simulink model "case4"  (R2024b)
settings: Solver=FixedStepAuto  StartTime=0  StopTime=1  FixedStep=1e-7  RelTol=1e-3
values from neighbouring files (symbols this model uses):
  SG_D_1_D = 0.01056    [IEEE9_case_parameters.m]    (also in case1_parameters.m; case2_parameters.m; case3_parameters.m; case4_parameters.m)
  SG_D_1_EnableSaturation = 0    [IEEE9_case_parameters.m]    (also in case1_parameters.m; case2_parameters.m; case3_parameters.m; case4_parameters.m)
  SG_D_1_f0 = 60    [IEEE9_case_parameters.m]    (also in case1_parameters.m; case2_parameters.m; case3_parameters.m; case4_parameters.m)
  SG_D_1_H = 7.5    [IEEE9_case_parameters.m]    (also in case1_parameters.m; case2_parameters.m; case3_parameters.m; case4_parameters.m)
  SG_D_1_K_A = 20    [IEEE9_case_parameters.m]    (also in case1_parameters.m; case2_parameters.m; case3_parameters.m; case4_parameters.m)
  SG_D_1_K_E = 1.000000e+1    (= 10)    [IEEE9_case_parameters.m]    (also in case1_parameters.m; case2_parameters.m; case3_parameters.m; case4_parameters.m)
  SG_D_1_K_F = 2.363    [IEEE9_case_parameters.m]    (also in case1_parameters.m; case2_parameters.m; case3_parameters.m; case4_parameters.m)
  SG_D_1_K_s = 0.5    [IEEE9_case_parameters.m]    (also in case1_parameters.m = 5; case2_parameters.m = 5; case3_parameters.m = 5; case4_parameters.m = 5)
  SG_D_1_R_a = 0.001088    [IEEE9_case_parameters.m]    (also in case1_parameters.m; case2_parameters.m; case3_parameters.m; case4_parameters.m)
  SG_D_1_S_A = 1    [IEEE9_case_parameters.m]    (also in case1_parameters.m; case2_parameters.m; case3_parameters.m; case4_parameters.m)
  SG_D_1_S_B = 0.103    [IEEE9_case_parameters.m]    (also in case1_parameters.m; case2_parameters.m; case3_parameters.m; case4_parameters.m)
  SG_D_1_S_N = 10.659857    [IEEE9_case_parameters.m]    (also in case1_parameters.m; case2_parameters.m; case3_parameters.m; case4_parameters.m)
  SG_D_1_SpeedPara = 200    [IEEE9_case_parameters.m]    (also in case1_parameters.m; case2_parameters.m; case3_parameters.m; case4_parameters.m)
  SG_D_1_T_0 = 0.720173    [IEEE9_case_parameters.m]    (also in case1_parameters.m = 0.755522; case2_parameters.m = 0.808931; case3_parameters.m = 0.869402; case4_parameters.m = 0.729316)
  SG_D_1_T_1 = 0.3    [IEEE9_case_parameters.m]    (also in case1_parameters.m; case2_parameters.m; case3_parameters.m; case4_parameters.m)
  SG_D_1_T_2 = 0.05    [IEEE9_case_parameters.m]    (also in case1_parameters.m; case2_parameters.m; case3_parameters.m; case4_parameters.m)
  SG_D_1_T_3 = 0.02    [IEEE9_case_parameters.m]    (also in case1_parameters.m; case2_parameters.m; case3_parameters.m; case4_parameters.m)
  SG_D_1_T_4 = 0.005    [IEEE9_case_parameters.m]    (also in case1_parameters.m; case2_parameters.m; case3_parameters.m; case4_parameters.m)
  SG_D_1_T_A = 0.02    [IEEE9_case_parameters.m]    (also in case1_parameters.m; case2_parameters.m; case3_parameters.m; case4_parameters.m)
  SG_D_1_T_dd = 8.000000e+0    (= 8)    [IEEE9_case_parameters.m]    (also in case1_parameters.m; case2_parameters.m; case3_parameters.m; case4_parameters.m)
  SG_D_1_T_ddd = 0.04    [IEEE9_case_parameters.m]    (also in case1_parameters.m; case2_parameters.m; case3_parameters.m; case4_parameters.m)
  SG_D_1_T_E = 0.314    [IEEE9_case_parameters.m]    (also in case1_parameters.m; case2_parameters.m; case3_parameters.m; case4_parameters.m)
  SG_D_1_T_F = 0.35    [IEEE9_case_parameters.m]    (also in case1_parameters.m; case2_parameters.m; case3_parameters.m; case4_parameters.m)
  SG_D_1_T_qd = 0.8    [IEEE9_case_parameters.m]    (also in case1_parameters.m; case2_parameters.m; case3_parameters.m; case4_parameters.m)
  SG_D_1_T_qdd = 0.02    [IEEE9_case_parameters.m]    (also in case1_parameters.m; case2_parameters.m; case3_parameters.m; case4_parameters.m)
  SG_D_1_T_speed = 0.1    [IEEE9_case_parameters.m]    (also in case1_parameters.m = 200; case2_parameters.m = 200; case3_parameters.m = 200; case4_parameters.m = 200)
  SG_D_1_T_w = 0.5    [IEEE9_case_parameters.m]    (also in case1_parameters.m; case2_parameters.m; case3_parameters.m; case4_parameters.m)
  SG_D_1_V_ref = 1.990276    [IEEE9_case_parameters.m]    (also in case1_parameters.m = 2.042296; case2_parameters.m = 2.051388; case3_parameters.m = 2.089584; case4_parameters.m = 2.01845)
  SG_D_1_w_ref = 376.991118    [IEEE9_case_parameters.m]    (also in case1_parameters.m; case2_parameters.m; case3_parameters.m; case4_parameters.m)
  SG_D_1_wb = 6.000000e+1    (= 60)    [IEEE9_case_parameters.m]    (also in case1_parameters.m; case2_parameters.m; case3_parameters.m; case4_parameters.m)
  SG_D_1_x_d = 1.9    [IEEE9_case_parameters.m]    (also in case1_parameters.m; case2_parameters.m; case3_parameters.m; case4_parameters.m)
  SG_D_1_x_dd = 0.302    [IEEE9_case_parameters.m]    (also in case1_parameters.m; case2_parameters.m; case3_parameters.m; case4_parameters.m)
  SG_D_1_x_ddd = 0.204    [IEEE9_case_parameters.m]    (also in case1_parameters.m; case2_parameters.m; case3_parameters.m; case4_parameters.m)
  SG_D_1_x_l = 0.05    [IEEE9_case_parameters.m]    (also in case1_parameters.m; case2_parameters.m; case3_parameters.m; case4_parameters.m)
  SG_D_1_x_q = 1.3    [IEEE9_case_parameters.m]    (also in case1_parameters.m; case2_parameters.m; case3_parameters.m; case4_parameters.m)
  SG_D_1_x_qd = 0.5    [IEEE9_case_parameters.m]    (also in case1_parameters.m; case2_parameters.m; case3_parameters.m; case4_parameters.m)
  SG_D_1_x_qdd = 0.3    [IEEE9_case_parameters.m]    (also in case1_parameters.m; case2_parameters.m; case3_parameters.m; case4_parameters.m)
  SG_D_2_D = 0.02    [IEEE9_case_parameters.m]    (also in case1_parameters.m; case2_parameters.m; case3_parameters.m; case4_parameters.m)
  SG_D_2_EnableSaturation = 0    [IEEE9_case_parameters.m]    (also in case1_parameters.m; case2_parameters.m; case3_parameters.m; case4_parameters.m)
  SG_D_2_f0 = 60    [IEEE9_case_parameters.m]    (also in case1_parameters.m; case2_parameters.m; case3_parameters.m; case4_parameters.m)
  SG_D_2_H = 8.000000e+0    (= 8)    [IEEE9_case_parameters.m]    (also in case1_parameters.m; case2_parameters.m; case3_parameters.m; case4_parameters.m)
  SG_D_2_K_A = 20    [IEEE9_case_parameters.m]    (also in case1_parameters.m; case2_parameters.m; case3_parameters.m; case4_parameters.m)
  SG_D_2_K_E = 1.000000e+1    (= 10)    [IEEE9_case_parameters.m]    (also in case1_parameters.m; case2_parameters.m; case3_parameters.m; case4_parameters.m)
  SG_D_2_K_F = 2.363    [IEEE9_case_parameters.m]    (also in case1_parameters.m; case2_parameters.m; case3_parameters.m; case4_parameters.m)
  SG_D_2_K_s = 0.5    [IEEE9_case_parameters.m]    (also in case1_parameters.m = 4; case2_parameters.m = 4; case3_parameters.m = 4; case4_parameters.m = 4)
  SG_D_2_R_a = 0.001088    [IEEE9_case_parameters.m]    (also in case1_parameters.m; case2_parameters.m; case3_parameters.m; case4_parameters.m)
  SG_D_2_S_A = 1    [IEEE9_case_parameters.m]    (also in case1_parameters.m; case2_parameters.m; case3_parameters.m; case4_parameters.m)
  SG_D_2_S_B = 0.103    [IEEE9_case_parameters.m]    (also in case1_parameters.m; case2_parameters.m; case3_parameters.m; case4_parameters.m)
  SG_D_2_S_N = 10.659857    [IEEE9_case_parameters.m]    (also in case1_parameters.m; case2_parameters.m; case3_parameters.m; case4_parameters.m)
  SG_D_2_SpeedPara = 200    [IEEE9_case_parameters.m]    (also in case1_parameters.m; case2_parameters.m; case3_parameters.m; case4_parameters.m)
  SG_D_2_T_0 = 1.632913    [IEEE9_case_parameters.m]    (also in case1_parameters.m = 1.632925; case2_parameters.m = 1.632915; case3_parameters.m = 1.632914; case4_parameters.m = 1.632927)
  SG_D_2_T_1 = 0.2    [IEEE9_case_parameters.m]    (also in case1_parameters.m; case2_parameters.m; case3_parameters.m; case4_parameters.m)
  SG_D_2_T_2 = 0.05    [IEEE9_case_parameters.m]    (also in case1_parameters.m; case2_parameters.m; case3_parameters.m; case4_parameters.m)
  SG_D_2_T_3 = 0.02    [IEEE9_case_parameters.m]    (also in case1_parameters.m; case2_parameters.m; case3_parameters.m; case4_parameters.m)
  SG_D_2_T_4 = 0.005    [IEEE9_case_parameters.m]    (also in case1_parameters.m; case2_parameters.m; case3_parameters.m; case4_parameters.m)
  SG_D_2_T_A = 0.02    [IEEE9_case_parameters.m]    (also in case1_parameters.m; case2_parameters.m; case3_parameters.m; case4_parameters.m)
  SG_D_2_T_dd = 7.9    [IEEE9_case_parameters.m]    (also in case1_parameters.m; case2_parameters.m; case3_parameters.m; case4_parameters.m)
  SG_D_2_T_ddd = 0.04    [IEEE9_case_parameters.m]    (also in case1_parameters.m; case2_parameters.m; case3_parameters.m; case4_parameters.m)
  SG_D_2_T_E = 0.314    [IEEE9_case_parameters.m]    (also in case1_parameters.m; case2_parameters.m; case3_parameters.m; case4_parameters.m)
  SG_D_2_T_F = 0.35    [IEEE9_case_parameters.m]    (also in case1_parameters.m; case2_parameters.m; case3_parameters.m; case4_parameters.m)
  SG_D_2_T_qd = 0.8    [IEEE9_case_parameters.m]    (also in case1_parameters.m; case2_parameters.m; case3_parameters.m; case4_parameters.m)
  SG_D_2_T_qdd = 0.015    [IEEE9_case_parameters.m]    (also in case1_parameters.m; case2_parameters.m; case3_parameters.m; case4_parameters.m)
  SG_D_2_T_speed = 0.1    [IEEE9_case_parameters.m]    (also in case1_parameters.m = 150; case2_parameters.m = 150; case3_parameters.m = 150; case4_parameters.m = 150)
  SG_D_2_T_w = 0.35    [IEEE9_case_parameters.m]    (also in case1_parameters.m; case2_parameters.m; case3_parameters.m; case4_parameters.m)
  SG_D_2_V_ref = 2.58547    [IEEE9_case_parameters.m]    (also in case1_parameters.m = 2.597896; case2_parameters.m = 2.587136; case3_parameters.m = 2.586042; case4_parameters.m = 2.599679)
  SG_D_2_w_ref = 376.991118    [IEEE9_case_parameters.m]    (also in case1_parameters.m; case2_parameters.m; case3_parameters.m; case4_parameters.m)
  SG_D_2_wb = 6.000000e+1    (= 60)    [IEEE9_case_parameters.m]    (also in case1_parameters.m; case2_parameters.m; case3_parameters.m; case4_parameters.m)
  SG_D_2_x_d = 1.8    [IEEE9_case_parameters.m]    (also in case1_parameters.m; case2_parameters.m; case3_parameters.m; case4_parameters.m)
  SG_D_2_x_dd = 0.302    [IEEE9_case_parameters.m]    (also in case1_parameters.m; case2_parameters.m; case3_parameters.m; case4_parameters.m)
  SG_D_2_x_ddd = 0.204    [IEEE9_case_parameters.m]    (also in case1_parameters.m; case2_parameters.m; case3_parameters.m; case4_parameters.m)
  SG_D_2_x_l = 0.05    [IEEE9_case_parameters.m]    (also in case1_parameters.m; case2_parameters.m; case3_parameters.m; case4_parameters.m)
  SG_D_2_x_q = 1.25    [IEEE9_case_parameters.m]    (also in case1_parameters.m; case2_parameters.m; case3_parameters.m; case4_parameters.m)
  SG_D_2_x_qd = 0.5    [IEEE9_case_parameters.m]    (also in case1_parameters.m; case2_parameters.m; case3_parameters.m; case4_parameters.m)
  SG_D_2_x_qdd = 0.3    [IEEE9_case_parameters.m]    (also in case1_parameters.m; case2_parameters.m; case3_parameters.m; case4_parameters.m)
  SG_D_3_D = 0.02    [IEEE9_case_parameters.m]    (also in case1_parameters.m; case2_parameters.m; case3_parameters.m; case4_parameters.m)
  SG_D_3_EnableSaturation = 0    [IEEE9_case_parameters.m]    (also in case1_parameters.m; case2_parameters.m; case3_parameters.m; case4_parameters.m)
  SG_D_3_f0 = 60    [IEEE9_case_parameters.m]    (also in case1_parameters.m; case2_parameters.m; case3_parameters.m; case4_parameters.m)
  SG_D_3_H = 7.7    [IEEE9_case_parameters.m]    (also in case1_parameters.m; case2_parameters.m; case3_parameters.m; case4_parameters.m)
  SG_D_3_K_A = 20    [IEEE9_case_parameters.m]    (also in case1_parameters.m; case2_parameters.m; case3_parameters.m; case4_parameters.m)
  SG_D_3_K_E = 1.000000e+1    (= 10)    [IEEE9_case_parameters.m]    (also in case1_parameters.m; case2_parameters.m; case3_parameters.m; case4_parameters.m)
  SG_D_3_K_F = 2.363    [IEEE9_case_parameters.m]    (also in case1_parameters.m; case2_parameters.m; case3_parameters.m; case4_parameters.m)
  SG_D_3_K_s = 0.2    [IEEE9_case_parameters.m]    (also in case1_parameters.m = 2; case2_parameters.m = 2; case3_parameters.m = 2; case4_parameters.m = 2)
  SG_D_3_R_a = 0.001088    [IEEE9_case_parameters.m]    (also in case1_parameters.m; case2_parameters.m; case3_parameters.m; case4_parameters.m)
  SG_D_3_S_A = 1    [IEEE9_case_parameters.m]    (also in case1_parameters.m; case2_parameters.m; case3_parameters.m; case4_parameters.m)
  SG_D_3_S_B = 0.103    [IEEE9_case_parameters.m]    (also in case1_parameters.m; case2_parameters.m; case3_parameters.m; case4_parameters.m)
  SG_D_3_S_N = 10.659857    [IEEE9_case_parameters.m]    (also in case1_parameters.m; case2_parameters.m; case3_parameters.m; case4_parameters.m)
  SG_D_3_SpeedPara = 200    [IEEE9_case_parameters.m]    (also in case1_parameters.m; case2_parameters.m; case3_parameters.m; case4_parameters.m)
  SG_D_3_T_0 = 0.850788    [IEEE9_case_parameters.m]    (also in case1_parameters.m = 0.850786; case2_parameters.m = 0.850787; case3_parameters.m; case4_parameters.m = 0.850786)
  SG_D_3_T_1 = 0.2    [IEEE9_case_parameters.m]    (also in case1_parameters.m; case2_parameters.m; case3_parameters.m; case4_parameters.m)
  SG_D_3_T_2 = 0.05    [IEEE9_case_parameters.m]    (also in case1_parameters.m; case2_parameters.m; case3_parameters.m; case4_parameters.m)
  SG_D_3_T_3 = 0.02    [IEEE9_case_parameters.m]    (also in case1_parameters.m; case2_parameters.m; case3_parameters.m; case4_parameters.m)
  SG_D_3_T_4 = 0.005    [IEEE9_case_parameters.m]    (also in case1_parameters.m; case2_parameters.m; case3_parameters.m; case4_parameters.m)
  SG_D_3_T_A = 0.02    [IEEE9_case_parameters.m]    (also in case1_parameters.m; case2_parameters.m; case3_parameters.m; case4_parameters.m)
  SG_D_3_T_dd = 8.1    [IEEE9_case_parameters.m]    (also in case1_parameters.m; case2_parameters.m; case3_parameters.m; case4_parameters.m)
  SG_D_3_T_ddd = 0.04    [IEEE9_case_parameters.m]    (also in case1_parameters.m; case2_parameters.m; case3_parameters.m; case4_parameters.m)
  SG_D_3_T_E = 0.314    [IEEE9_case_parameters.m]    (also in case1_parameters.m; case2_parameters.m; case3_parameters.m; case4_parameters.m)
  SG_D_3_T_F = 0.35    [IEEE9_case_parameters.m]    (also in case1_parameters.m; case2_parameters.m; case3_parameters.m; case4_parameters.m)
  SG_D_3_T_qd = 0.8    [IEEE9_case_parameters.m]    (also in case1_parameters.m; case2_parameters.m; case3_parameters.m; case4_parameters.m)
  SG_D_3_T_qdd = 0.015    [IEEE9_case_parameters.m]    (also in case1_parameters.m; case2_parameters.m; case3_parameters.m; case4_parameters.m)
  SG_D_3_T_speed = 0.1    [IEEE9_case_parameters.m]    (also in case1_parameters.m = 180; case2_parameters.m = 180; case3_parameters.m = 180; case4_parameters.m = 180)
  SG_D_3_T_w = 0.4    [IEEE9_case_parameters.m]    (also in case1_parameters.m; case2_parameters.m; case3_parameters.m; case4_parameters.m)
  SG_D_3_V_ref = 1.892727    [IEEE9_case_parameters.m]    (also in case1_parameters.m = 1.906439; case2_parameters.m = 1.895535; case3_parameters.m = 1.892105; case4_parameters.m = 1.906598)
  SG_D_3_w_ref = 376.991118    [IEEE9_case_parameters.m]    (also in case1_parameters.m; case2_parameters.m; case3_parameters.m; case4_parameters.m)
  SG_D_3_wb = 6.000000e+1    (= 60)    [IEEE9_case_parameters.m]    (also in case1_parameters.m; case2_parameters.m; case3_parameters.m; case4_parameters.m)
  SG_D_3_x_d = 1.85    [IEEE9_case_parameters.m]    (also in case1_parameters.m; case2_parameters.m; case3_parameters.m; case4_parameters.m)
  SG_D_3_x_dd = 0.302    [IEEE9_case_parameters.m]    (also in case1_parameters.m; case2_parameters.m; case3_parameters.m; case4_parameters.m)
  SG_D_3_x_ddd = 0.204    [IEEE9_case_parameters.m]    (also in case1_parameters.m; case2_parameters.m; case3_parameters.m; case4_parameters.m)
  SG_D_3_x_l = 0.05    [IEEE9_case_parameters.m]    (also in case1_parameters.m; case2_parameters.m; case3_parameters.m; case4_parameters.m)
  SG_D_3_x_q = 1.2    [IEEE9_case_parameters.m]    (also in case1_parameters.m; case2_parameters.m; case3_parameters.m; case4_parameters.m)
  SG_D_3_x_qd = 0.5    [IEEE9_case_parameters.m]    (also in case1_parameters.m; case2_parameters.m; case3_parameters.m; case4_parameters.m)
  SG_D_3_x_qdd = 0.3    [IEEE9_case_parameters.m]    (also in case1_parameters.m; case2_parameters.m; case3_parameters.m; case4_parameters.m)
(part 2 of 12)

== system case4/SG_D_2 ==
  v_d_SG_D_2 : Inport
  v_q_SG_D_2 : Inport  Port=2
  E_fd_SG_D_2 : Integrator  InitialCondition=3.199358804894044
  Px_1_SG_D_2 : Integrator  InitialCondition=0.0
  Px_2_SG_D_2 : Integrator  InitialCondition=0.0
  Px_3_SG_D_2 : Integrator  InitialCondition=-1.0252237820631645e-24
  R_f_SG_D_2 : Integrator  InitialCondition=21.60024244561322
  T_e_SG_D_2_block : Subsystem
  T_m_SG_D_2 : Integrator  InitialCondition=1.632927067566547
  V_f_SG_D_2 : Integrator  InitialCondition=31.993588048940442
  d_E_fd_SG_D_2_block : Subsystem
  d_Px_1_SG_D_2_block : Subsystem
  d_Px_2_SG_D_2_block : Subsystem
  d_Px_3_SG_D_2_block : Subsystem
  d_R_f_SG_D_2_block : Subsystem
  d_T_m_SG_D_2_block : Subsystem
  d_V_f_SG_D_2_block : Subsystem
  d_psi_1d_SG_D_2_block : Subsystem
  d_psi_d_SG_D_2_block : Subsystem
  d_psi_fd_SG_D_2_block : Subsystem
  d_psi_gq_SG_D_2_block : Subsystem
  d_psi_kq_SG_D_2_block : Subsystem
  d_psi_q_SG_D_2_block : Subsystem
  d_theta_SG_D_2_block : Subsystem
  d_w_SG_D_2_block : Subsystem
  i_d_SG_D_2_block : Subsystem
  i_q_SG_D_2_block : Subsystem
  psi_1d_SG_D_2 : Integrator  InitialCondition=0.5921734460690405
  psi_d_SG_D_2 : Integrator  InitialCondition=0.5176824358168975
  psi_fd_SG_D_2 : Integrator  InitialCondition=0.9676081377398411
  psi_gq_SG_D_2 : Integrator  InitialCondition=0.514587004954726
  psi_kq_SG_D_2 : Integrator  InitialCondition=-0.8233392079275615
  psi_q_SG_D_2 : Integrator  InitialCondition=-0.8576450082578766
  theta_SG_D_2 : Integrator  InitialCondition=1.203497719672738
  theta_SG_D_2_out_block : Subsystem
  w_SG_D_2 : Integrator  InitialCondition=376.99111843077515
  w_SG_D_2_out_block : Subsystem
  i_d_SG_D_2 : Outport
  i_q_SG_D_2 : Outport  Port=2
  T_e_SG_D_2 : Outport  Port=3
  w_SG_D_2_out : Outport  Port=4
  theta_SG_D_2_out : Outport  Port=5
  wires:
  T_e_SG_D_2_block/1(Blockout_T_e_SG_D_2_aeb34) -> T_e_SG_D_2/1
  d_Px_2_SG_D_2_block/1(Blockout_d_Px_2_SG_D_2_a31a2) -> Px_2_SG_D_2/1
  d_T_m_SG_D_2_block/1(Blockout_d_T_m_SG_D_2_16fb0) -> T_m_SG_D_2/1
  w_SG_D_2/1 -> d_w_SG_D_2_block/1(State_w_SG_D_2_24507), d_psi_d_SG_D_2_block/9(State_w_SG_D_2_062a2), d_V_f_SG_D_2_block/13(State_w_SG_D_2_1f752), d_psi_q_SG_D_2_block/9(State_w_SG_D_2_85500), d_T_m_SG_D_2_block/1(State_w_SG_D_2_20fb2), d_theta_SG_D_2_block/1(State_w_SG_D_2_83554), d_Px_2_SG_D_2_block/4(State_w_SG_D_2_251c8), d_Px_3_SG_D_2_block/6(State_w_SG_D_2_cceda), d_Px_1_SG_D_2_block/2(State_w_SG_D_2_89096), w_SG_D_2_out_block/1(State_w_SG_D_2_49837), d_V_f_SG_D_2_block/8(State_w_SG_D_2_d8cc8)
  psi_q_SG_D_2/1 -> d_psi_d_SG_D_2_block/8(State_psi_q_SG_D_2_4ef81), d_psi_gq_SG_D_2_block/6(State_psi_q_SG_D_2_42d41), d_psi_gq_SG_D_2_block/9(State_psi_q_SG_D_2_df93d), d_psi_q_SG_D_2_block/3(State_psi_q_SG_D_2_7ccc9), d_psi_kq_SG_D_2_block/5(State_psi_q_SG_D_2_06ac6), d_w_SG_D_2_block/6(State_psi_q_SG_D_2_486c0), d_w_SG_D_2_block/7(State_psi_q_SG_D_2_c0a51), i_d_SG_D_2_block/3(State_psi_q_SG_D_2_d9bdd), i_q_SG_D_2_block/3(State_psi_q_SG_D_2_089b8), d_V_f_SG_D_2_block/7(State_psi_q_SG_D_2_113af), T_e_SG_D_2_block/4(State_psi_q_SG_D_2_38137), T_e_SG_D_2_block/5(State_psi_q_SG_D_2_ed317), d_V_f_SG_D_2_block/11(State_psi_q_SG_D_2_905ca)
  w_SG_D_2_out_block/1(Blockout_w_SG_D_2_out_2aeb7) -> w_SG_D_2_out/1
  T_m_SG_D_2/1 -> d_T_m_SG_D_2_block/2(State_T_m_SG_D_2_247d7), d_w_SG_D_2_block/2(State_T_m_SG_D_2_a1094)
  d_theta_SG_D_2_block/1(Blockout_d_theta_SG_D_2_36a6f) -> theta_SG_D_2/1
  d_Px_1_SG_D_2_block/1(Blockout_d_Px_1_SG_D_2_f7300) -> Px_1_SG_D_2/1
  d_Px_3_SG_D_2_block/1(Blockout_d_Px_3_SG_D_2_a07c3) -> Px_3_SG_D_2/1
  Px_2_SG_D_2/1 -> d_Px_2_SG_D_2_block/1(State_Px_2_SG_D_2_0c5e7), d_Px_3_SG_D_2_block/2(State_Px_2_SG_D_2_117c1), d_Px_3_SG_D_2_block/3(State_Px_2_SG_D_2_e0625)
  theta_SG_D_2/1 -> d_psi_d_SG_D_2_block/7(State_theta_SG_D_2_7f4d5), i_d_SG_D_2_block/8(State_theta_SG_D_2_c3678), i_q_SG_D_2_block/4(State_theta_SG_D_2_9d528), d_psi_q_SG_D_2_block/7(State_theta_SG_D_2_47b3e), i_q_SG_D_2_block/8(State_theta_SG_D_2_f85ec), i_d_SG_D_2_block/4(State_theta_SG_D_2_d89e5), theta_SG_D_2_out_block/1(State_theta_SG_D_2_ce1d4), d_psi_q_SG_D_2_block/5(State_theta_SG_D_2_14fc9), d_psi_d_SG_D_2_block/5(State_theta_SG_D_2_f56a2)
  i_d_SG_D_2_block/1(Blockout_i_d_SG_D_2_51594) -> i_d_SG_D_2/1
  psi_d_SG_D_2/1 -> d_psi_fd_SG_D_2_block/6(State_psi_d_SG_D_2_a4384), d_psi_fd_SG_D_2_block/9(State_psi_d_SG_D_2_a1f54), d_psi_d_SG_D_2_block/2(State_psi_d_SG_D_2_af81e), d_psi_q_SG_D_2_block/8(State_psi_d_SG_D_2_a9787), d_psi_1d_SG_D_2_block/4(State_psi_d_SG_D_2_8f652), d_w_SG_D_2_block/9(State_psi_d_SG_D_2_07c04), d_w_SG_D_2_block/3(State_psi_d_SG_D_2_9e36d), d_V_f_SG_D_2_block/5(State_psi_d_SG_D_2_88c50), d_V_f_SG_D_2_block/12(State_psi_d_SG_D_2_b6804), i_d_SG_D_2_block/6(State_psi_d_SG_D_2_cc06c), i_q_SG_D_2_block/6(State_psi_d_SG_D_2_1475e), T_e_SG_D_2_block/1(State_psi_d_SG_D_2_11756), T_e_SG_D_2_block/7(State_psi_d_SG_D_2_9e42d)
  v_d_SG_D_2/1 -> d_psi_d_SG_D_2_block/4(Input_v_d_SG_D_2_dee58), d_psi_q_SG_D_2_block/4(Input_v_d_SG_D_2_9a544)
  d_V_f_SG_D_2_block/1(Blockout_d_V_f_SG_D_2_08704) -> V_f_SG_D_2/1
  v_q_SG_D_2/1 -> d_psi_d_SG_D_2_block/6(Input_v_q_SG_D_2_fe918), d_psi_q_SG_D_2_block/6(Input_v_q_SG_D_2_bd14d)
  psi_fd_SG_D_2/1 -> d_psi_fd_SG_D_2_block/2(State_psi_fd_SG_D_2_402f0), d_psi_fd_SG_D_2_block/7(State_psi_fd_SG_D_2_f7400), d_psi_fd_SG_D_2_block/4(State_psi_fd_SG_D_2_f381f), d_psi_d_SG_D_2_block/3(State_psi_fd_SG_D_2_c88a6), d_psi_fd_SG_D_2_block/10(State_psi_fd_SG_D_2_88820), d_w_SG_D_2_block/10(State_psi_fd_SG_D_2_cf8a3), d_psi_1d_SG_D_2_block/2(State_psi_fd_SG_D_2_d4a3d), d_V_f_SG_D_2_block/6(State_psi_fd_SG_D_2_5ba3e), d_psi_1d_SG_D_2_block/5(State_psi_fd_SG_D_2_2139b), i_d_SG_D_2_block/7(State_psi_fd_SG_D_2_3594a), i_q_SG_D_2_block/7(State_psi_fd_SG_D_2_02c56), T_e_SG_D_2_block/8(State_psi_fd_SG_D_2_0e9d9)
  psi_1d_SG_D_2/1 -> d_psi_fd_SG_D_2_block/3(State_psi_1d_SG_D_2_343a2), d_psi_fd_SG_D_2_block/5(State_psi_1d_SG_D_2_7e680), d_psi_fd_SG_D_2_block/8(State_psi_1d_SG_D_2_84c2e), d_psi_d_SG_D_2_block/1(State_psi_1d_SG_D_2_e94c1), d_psi_1d_SG_D_2_block/1(State_psi_1d_SG_D_2_89b76), d_psi_1d_SG_D_2_block/3(State_psi_1d_SG_D_2_48a12), d_V_f_SG_D_2_block/4(State_psi_1d_SG_D_2_6a683), d_w_SG_D_2_block/8(State_psi_1d_SG_D_2_8ca6f), i_q_SG_D_2_block/5(State_psi_1d_SG_D_2_35b9d), i_d_SG_D_2_block/5(State_psi_1d_SG_D_2_5ca32), T_e_SG_D_2_block/6(State_psi_1d_SG_D_2_6920c)
  psi_kq_SG_D_2/1 -> d_psi_q_SG_D_2_block/2(State_psi_kq_SG_D_2_849d4), d_psi_gq_SG_D_2_block/3(State_psi_kq_SG_D_2_628c0), d_psi_gq_SG_D_2_block/5(State_psi_kq_SG_D_2_b8dc9), d_psi_gq_SG_D_2_block/8(State_psi_kq_SG_D_2_bcc03), d_V_f_SG_D_2_block/10(State_psi_kq_SG_D_2_52314), d_psi_kq_SG_D_2_block/4(State_psi_kq_SG_D_2_92652), d_psi_kq_SG_D_2_block/2(State_psi_kq_SG_D_2_02eb9), i_d_SG_D_2_block/2(State_psi_kq_SG_D_2_4dc54), i_q_SG_D_2_block/2(State_psi_kq_SG_D_2_4278f), T_e_SG_D_2_block/3(State_psi_kq_SG_D_2_da24b), d_w_SG_D_2_block/5(State_psi_kq_SG_D_2_3a13f)
  Px_1_SG_D_2/1 -> d_Px_3_SG_D_2_block/5(State_Px_1_SG_D_2_7e22a), d_Px_2_SG_D_2_block/3(State_Px_1_SG_D_2_9542b), d_Px_1_SG_D_2_block/1(State_Px_1_SG_D_2_ffc5d), d_Px_3_SG_D_2_block/4(State_Px_1_SG_D_2_71ec3), d_Px_2_SG_D_2_block/2(State_Px_1_SG_D_2_d066c)
  psi_gq_SG_D_2/1 -> d_psi_q_SG_D_2_block/1(State_psi_gq_SG_D_2_e6c3e), d_psi_gq_SG_D_2_block/1(State_psi_gq_SG_D_2_ab3da), d_psi_gq_SG_D_2_block/2(State_psi_gq_SG_D_2_60145), d_psi_kq_SG_D_2_block/3(State_psi_gq_SG_D_2_77eb3), d_w_SG_D_2_block/4(State_psi_gq_SG_D_2_52eb9), d_V_f_SG_D_2_block/9(State_psi_gq_SG_D_2_851e3), i_d_SG_D_2_block/1(State_psi_gq_SG_D_2_b50ef), T_e_SG_D_2_block/2(State_psi_gq_SG_D_2_3103f), i_q_SG_D_2_block/1(State_psi_gq_SG_D_2_b06e0), d_psi_gq_SG_D_2_block/7(State_psi_gq_SG_D_2_d38f4), d_psi_kq_SG_D_2_block/1(State_psi_gq_SG_D_2_8d7c7), d_psi_gq_SG_D_2_block/4(State_psi_gq_SG_D_2_262a5)
  d_R_f_SG_D_2_block/1(Blockout_d_R_f_SG_D_2_5255c) -> R_f_SG_D_2/1
  d_psi_1d_SG_D_2_block/1(Blockout_d_psi_1d_SG_D_2_0e78a) -> psi_1d_SG_D_2/1
  i_q_SG_D_2_block/1(Blockout_i_q_SG_D_2_f7c08) -> i_q_SG_D_2/1
  R_f_SG_D_2/1 -> d_V_f_SG_D_2_block/2(State_R_f_SG_D_2_2b1aa), d_R_f_SG_D_2_block/2(State_R_f_SG_D_2_f9839)
  theta_SG_D_2_out_block/1(Blockout_theta_SG_D_2_out_e80c4) -> theta_SG_D_2_out/1
  d_w_SG_D_2_block/1(Blockout_d_w_SG_D_2_310bb) -> w_SG_D_2/1
  d_psi_d_SG_D_2_block/1(Blockout_d_psi_d_SG_D_2_f1be8) -> psi_d_SG_D_2/1
  d_psi_q_SG_D_2_block/1(Blockout_d_psi_q_SG_D_2_4e8af) -> psi_q_SG_D_2/1
  d_psi_kq_SG_D_2_block/1(Blockout_d_psi_kq_SG_D_2_5a47a) -> psi_kq_SG_D_2/1
  d_psi_gq_SG_D_2_block/1(Blockout_d_psi_gq_SG_D_2_5c396) -> psi_gq_SG_D_2/1
  V_f_SG_D_2/1 -> d_V_f_SG_D_2_block/14(State_V_f_SG_D_2_9fca1), d_E_fd_SG_D_2_block/2(State_V_f_SG_D_2_8bae1)
  Px_3_SG_D_2/1 -> d_V_f_SG_D_2_block/3(State_Px_3_SG_D_2_37027), d_Px_3_SG_D_2_block/1(State_Px_3_SG_D_2_1b144)
  d_E_fd_SG_D_2_block/1(Blockout_d_E_fd_SG_D_2_ce12b) -> E_fd_SG_D_2/1
  E_fd_SG_D_2/1 -> d_V_f_SG_D_2_block/1(State_E_fd_SG_D_2_a1ee9), d_R_f_SG_D_2_block/1(State_E_fd_SG_D_2_6574e), d_E_fd_SG_D_2_block/1(State_E_fd_SG_D_2_90b3d), d_psi_fd_SG_D_2_block/1(State_E_fd_SG_D_2_f08a6)
  d_psi_fd_SG_D_2_block/1(Blockout_d_psi_fd_SG_D_2_9880d) -> psi_fd_SG_D_2/1

== system case4/SG_D_3 ==
  v_d_SG_D_3 : Inport
  v_q_SG_D_3 : Inport  Port=2
  E_fd_SG_D_3 : Integrator  InitialCondition=1.8131955925748924
  Px_1_SG_D_3 : Integrator  InitialCondition=0.0
  Px_2_SG_D_3 : Integrator  InitialCondition=0.0
  Px_3_SG_D_3 : Integrator  InitialCondition=-4.454233030581895e-24
  R_f_SG_D_3 : Integrator  InitialCondition=12.241660529298489
  T_e_SG_D_3_block : Subsystem
  T_m_SG_D_3 : Integrator  InitialCondition=0.8507861821959377
  V_f_SG_D_3 : Integrator  InitialCondition=18.131955925748922
  d_E_fd_SG_D_3_block : Subsystem
  d_Px_1_SG_D_3_block : Subsystem
  d_Px_2_SG_D_3_block : Subsystem
  d_Px_3_SG_D_3_block : Subsystem
  d_R_f_SG_D_3_block : Subsystem
  d_T_m_SG_D_3_block : Subsystem
  d_V_f_SG_D_3_block : Subsystem
  d_psi_1d_SG_D_3_block : Subsystem
  d_psi_d_SG_D_3_block : Subsystem
  d_psi_fd_SG_D_3_block : Subsystem
  d_psi_gq_SG_D_3_block : Subsystem
  d_psi_kq_SG_D_3_block : Subsystem
  d_psi_q_SG_D_3_block : Subsystem
  d_theta_SG_D_3_block : Subsystem
  d_w_SG_D_3_block : Subsystem
  i_d_SG_D_3_block : Subsystem
  i_q_SG_D_3_block : Subsystem
  psi_1d_SG_D_3 : Integrator  InitialCondition=0.7270464685018727
  psi_d_SG_D_3 : Integrator  InitialCondition=0.6968756594998442
  psi_fd_SG_D_3 : Integrator  InitialCondition=0.8791073458720955
  psi_gq_SG_D_3 : Integrator  InitialCondition=0.41911384491220205
  psi_kq_SG_D_3 : Integrator  InitialCondition=-0.688544173784332
  psi_q_SG_D_3 : Integrator  InitialCondition=-0.7184808769923464
  theta_SG_D_3 : Integrator  InitialCondition=0.8867459021698747
  theta_SG_D_3_out_block : Subsystem
  w_SG_D_3 : Integrator  InitialCondition=376.99111843077515
  w_SG_D_3_out_block : Subsystem
  i_d_SG_D_3 : Outport
  i_q_SG_D_3 : Outport  Port=2
  T_e_SG_D_3 : Outport  Port=3
  w_SG_D_3_out : Outport  Port=4
  theta_SG_D_3_out : Outport  Port=5
  wires:
  d_Px_1_SG_D_3_block/1(Blockout_d_Px_1_SG_D_3_e0808) -> Px_1_SG_D_3/1
  w_SG_D_3/1 -> d_psi_q_SG_D_3_block/9(State_w_SG_D_3_e8c7b), d_w_SG_D_3_block/1(State_w_SG_D_3_b43dd), d_psi_d_SG_D_3_block/9(State_w_SG_D_3_7fa84), d_V_f_SG_D_3_block/13(State_w_SG_D_3_7eb7a), d_V_f_SG_D_3_block/8(State_w_SG_D_3_b47d2), d_theta_SG_D_3_block/1(State_w_SG_D_3_e7367), d_T_m_SG_D_3_block/1(State_w_SG_D_3_1fb5b), d_Px_1_SG_D_3_block/2(State_w_SG_D_3_8a56a), d_Px_2_SG_D_3_block/4(State_w_SG_D_3_c73de), d_Px_3_SG_D_3_block/6(State_w_SG_D_3_a3743), w_SG_D_3_out_block/1(State_w_SG_D_3_31263)
  d_T_m_SG_D_3_block/1(Blockout_d_T_m_SG_D_3_1d7fb) -> T_m_SG_D_3/1
  psi_kq_SG_D_3/1 -> d_psi_q_SG_D_3_block/2(State_psi_kq_SG_D_3_07912), d_psi_gq_SG_D_3_block/3(State_psi_kq_SG_D_3_7abd5), d_psi_kq_SG_D_3_block/2(State_psi_kq_SG_D_3_56f6b), d_psi_kq_SG_D_3_block/4(State_psi_kq_SG_D_3_5af45), d_V_f_SG_D_3_block/10(State_psi_kq_SG_D_3_0c819), d_w_SG_D_3_block/5(State_psi_kq_SG_D_3_1f8d8), i_d_SG_D_3_block/2(State_psi_kq_SG_D_3_67dcb), d_psi_gq_SG_D_3_block/5(State_psi_kq_SG_D_3_f6da0), i_q_SG_D_3_block/2(State_psi_kq_SG_D_3_30790), d_psi_gq_SG_D_3_block/8(State_psi_kq_SG_D_3_e83a4), T_e_SG_D_3_block/3(State_psi_kq_SG_D_3_5a7ef)
  d_Px_2_SG_D_3_block/1(Blockout_d_Px_2_SG_D_3_8eaa1) -> Px_2_SG_D_3/1
  R_f_SG_D_3/1 -> d_V_f_SG_D_3_block/2(State_R_f_SG_D_3_ced0f), d_R_f_SG_D_3_block/2(State_R_f_SG_D_3_7757e)
  w_SG_D_3_out_block/1(Blockout_w_SG_D_3_out_3b6ee) -> w_SG_D_3_out/1
  d_w_SG_D_3_block/1(Blockout_d_w_SG_D_3_07b1c) -> w_SG_D_3/1
  Px_1_SG_D_3/1 -> d_Px_3_SG_D_3_block/4(State_Px_1_SG_D_3_a976b), d_Px_2_SG_D_3_block/3(State_Px_1_SG_D_3_02523), d_Px_3_SG_D_3_block/5(State_Px_1_SG_D_3_b1c74), d_Px_2_SG_D_3_block/2(State_Px_1_SG_D_3_d6c88), d_Px_1_SG_D_3_block/1(State_Px_1_SG_D_3_e066f)
  d_theta_SG_D_3_block/1(Blockout_d_theta_SG_D_3_449e6) -> theta_SG_D_3/1
  d_Px_3_SG_D_3_block/1(Blockout_d_Px_3_SG_D_3_1ad82) -> Px_3_SG_D_3/1
  T_m_SG_D_3/1 -> d_T_m_SG_D_3_block/2(State_T_m_SG_D_3_64750), d_w_SG_D_3_block/2(State_T_m_SG_D_3_b0e8d)
  psi_gq_SG_D_3/1 -> d_psi_q_SG_D_3_block/1(State_psi_gq_SG_D_3_4bbcf), d_psi_gq_SG_D_3_block/1(State_psi_gq_SG_D_3_209b1), d_psi_gq_SG_D_3_block/2(State_psi_gq_SG_D_3_8cf71), d_psi_gq_SG_D_3_block/4(State_psi_gq_SG_D_3_9787e), d_psi_kq_SG_D_3_block/3(State_psi_gq_SG_D_3_442bf), d_w_SG_D_3_block/4(State_psi_gq_SG_D_3_9b74a), d_psi_gq_SG_D_3_block/7(State_psi_gq_SG_D_3_5ae7b), d_V_f_SG_D_3_block/9(State_psi_gq_SG_D_3_2ba50), i_d_SG_D_3_block/1(State_psi_gq_SG_D_3_033c6), d_psi_kq_SG_D_3_block/1(State_psi_gq_SG_D_3_8599d), i_q_SG_D_3_block/1(State_psi_gq_SG_D_3_d1da7), T_e_SG_D_3_block/2(State_psi_gq_SG_D_3_d6484)
  theta_SG_D_3/1 -> d_psi_d_SG_D_3_block/5(State_theta_SG_D_3_ca5af), d_psi_d_SG_D_3_block/7(State_theta_SG_D_3_ef297), d_psi_q_SG_D_3_block/5(State_theta_SG_D_3_91f0b), i_d_SG_D_3_block/4(State_theta_SG_D_3_0b2a8), i_d_SG_D_3_block/8(State_theta_SG_D_3_6b34c), i_q_SG_D_3_block/4(State_theta_SG_D_3_53a5b), i_q_SG_D_3_block/8(State_theta_SG_D_3_587af), theta_SG_D_3_out_block/1(State_theta_SG_D_3_e71d9), d_psi_q_SG_D_3_block/7(State_theta_SG_D_3_8654b)
  v_d_SG_D_3/1 -> d_psi_d_SG_D_3_block/4(Input_v_d_SG_D_3_d5357), d_psi_q_SG_D_3_block/4(Input_v_d_SG_D_3_64638)
  Px_2_SG_D_3/1 -> d_Px_2_SG_D_3_block/1(State_Px_2_SG_D_3_881a5), d_Px_3_SG_D_3_block/2(State_Px_2_SG_D_3_9dd6f), d_Px_3_SG_D_3_block/3(State_Px_2_SG_D_3_78cc5)
  v_q_SG_D_3/1 -> d_psi_d_SG_D_3_block/6(Input_v_q_SG_D_3_af468), d_psi_q_SG_D_3_block/6(Input_v_q_SG_D_3_99a28)
  psi_q_SG_D_3/1 -> d_psi_d_SG_D_3_block/8(State_psi_q_SG_D_3_aa699), d_psi_gq_SG_D_3_block/6(State_psi_q_SG_D_3_edd5e), d_psi_gq_SG_D_3_block/9(State_psi_q_SG_D_3_13abc), d_psi_kq_SG_D_3_block/5(State_psi_q_SG_D_3_8b826), d_w_SG_D_3_block/7(State_psi_q_SG_D_3_b15ed), d_V_f_SG_D_3_block/7(State_psi_q_SG_D_3_d1d11), d_psi_q_SG_D_3_block/3(State_psi_q_SG_D_3_50e34), d_V_f_SG_D_3_block/11(State_psi_q_SG_D_3_2a4c8), d_w_SG_D_3_block/6(State_psi_q_SG_D_3_897d4), T_e_SG_D_3_block/4(State_psi_q_SG_D_3_b778b), T_e_SG_D_3_block/5(State_psi_q_SG_D_3_ce48a), i_q_SG_D_3_block/3(State_psi_q_SG_D_3_debc5), i_d_SG_D_3_block/3(State_psi_q_SG_D_3_1df08)
  psi_d_SG_D_3/1 -> d_psi_fd_SG_D_3_block/9(State_psi_d_SG_D_3_7086f), d_psi_d_SG_D_3_block/2(State_psi_d_SG_D_3_f30ef), d_psi_q_SG_D_3_block/8(State_psi_d_SG_D_3_31b80), d_psi_1d_SG_D_3_block/4(State_psi_d_SG_D_3_4396d), d_w_SG_D_3_block/3(State_psi_d_SG_D_3_62c7d), d_w_SG_D_3_block/9(State_psi_d_SG_D_3_0d1fc), d_V_f_SG_D_3_block/5(State_psi_d_SG_D_3_92d1a), d_V_f_SG_D_3_block/12(State_psi_d_SG_D_3_fea1a), i_d_SG_D_3_block/6(State_psi_d_SG_D_3_e7225), d_psi_fd_SG_D_3_block/6(State_psi_d_SG_D_3_8f195), i_q_SG_D_3_block/6(State_psi_d_SG_D_3_fa48d), T_e_SG_D_3_block/1(State_psi_d_SG_D_3_77ae3), T_e_SG_D_3_block/7(State_psi_d_SG_D_3_80976)
  d_psi_kq_SG_D_3_block/1(Blockout_d_psi_kq_SG_D_3_86686) -> psi_kq_SG_D_3/1
  psi_1d_SG_D_3/1 -> d_psi_fd_SG_D_3_block/3(State_psi_1d_SG_D_3_83560), d_psi_fd_SG_D_3_block/5(State_psi_1d_SG_D_3_3b0bc), d_psi_fd_SG_D_3_block/8(State_psi_1d_SG_D_3_b04f8), d_psi_d_SG_D_3_block/1(State_psi_1d_SG_D_3_58f75), d_psi_1d_SG_D_3_block/3(State_psi_1d_SG_D_3_363e1), i_d_SG_D_3_block/5(State_psi_1d_SG_D_3_e063f), i_q_SG_D_3_block/5(State_psi_1d_SG_D_3_56eb2), d_V_f_SG_D_3_block/4(State_psi_1d_SG_D_3_0ab94), d_w_SG_D_3_block/8(State_psi_1d_SG_D_3_159bc), d_psi_1d_SG_D_3_block/1(State_psi_1d_SG_D_3_d1af3), T_e_SG_D_3_block/6(State_psi_1d_SG_D_3_88fd6)
  psi_fd_SG_D_3/1 -> d_psi_fd_SG_D_3_block/4(State_psi_fd_SG_D_3_42dbd), d_psi_fd_SG_D_3_block/10(State_psi_fd_SG_D_3_1261a), d_psi_d_SG_D_3_block/3(State_psi_fd_SG_D_3_ab767), d_psi_fd_SG_D_3_block/7(State_psi_fd_SG_D_3_830e0), d_psi_1d_SG_D_3_block/5(State_psi_fd_SG_D_3_d6b43), d_psi_1d_SG_D_3_block/2(State_psi_fd_SG_D_3_7715d), d_w_SG_D_3_block/10(State_psi_fd_SG_D_3_1e7f9), d_psi_fd_SG_D_3_block/2(State_psi_fd_SG_D_3_58a78), d_V_f_SG_D_3_block/6(State_psi_fd_SG_D_3_42f8c), i_d_SG_D_3_block/7(State_psi_fd_SG_D_3_2fd40), i_q_SG_D_3_block/7(State_psi_fd_SG_D_3_0b843), T_e_SG_D_3_block/8(State_psi_fd_SG_D_3_9b24b)
  theta_SG_D_3_out_block/1(Blockout_theta_SG_D_3_out_62f9d) -> theta_SG_D_3_out/1
  d_V_f_SG_D_3_block/1(Blockout_d_V_f_SG_D_3_c8238) -> V_f_SG_D_3/1
  d_psi_gq_SG_D_3_block/1(Blockout_d_psi_gq_SG_D_3_d606b) -> psi_gq_SG_D_3/1
  d_psi_q_SG_D_3_block/1(Blockout_d_psi_q_SG_D_3_12ce6) -> psi_q_SG_D_3/1
  d_R_f_SG_D_3_block/1(Blockout_d_R_f_SG_D_3_a651a) -> R_f_SG_D_3/1
  d_psi_d_SG_D_3_block/1(Blockout_d_psi_d_SG_D_3_4bd44) -> psi_d_SG_D_3/1
  i_d_SG_D_3_block/1(Blockout_i_d_SG_D_3_2136b) -> i_d_SG_D_3/1
  T_e_SG_D_3_block/1(Blockout_T_e_SG_D_3_61551) -> T_e_SG_D_3/1
  i_q_SG_D_3_block/1(Blockout_i_q_SG_D_3_16b07) -> i_q_SG_D_3/1
  d_psi_1d_SG_D_3_block/1(Blockout_d_psi_1d_SG_D_3_ecab5) -> psi_1d_SG_D_3/1
  Px_3_SG_D_3/1 -> d_Px_3_SG_D_3_block/1(State_Px_3_SG_D_3_a4ed4), d_V_f_SG_D_3_block/3(State_Px_3_SG_D_3_71c7e)
  V_f_SG_D_3/1 -> d_V_f_SG_D_3_block/14(State_V_f_SG_D_3_3c6cd), d_E_fd_SG_D_3_block/2(State_V_f_SG_D_3_0199b)
  d_E_fd_SG_D_3_block/1(Blockout_d_E_fd_SG_D_3_64aec) -> E_fd_SG_D_3/1
  E_fd_SG_D_3/1 -> d_V_f_SG_D_3_block/1(State_E_fd_SG_D_3_68a4f), d_R_f_SG_D_3_block/1(State_E_fd_SG_D_3_75620), d_E_fd_SG_D_3_block/1(State_E_fd_SG_D_3_21366), d_psi_fd_SG_D_3_block/1(State_E_fd_SG_D_3_ed17d)
  d_psi_fd_SG_D_3_block/1(Blockout_d_psi_fd_SG_D_3_1d4a8) -> psi_fd_SG_D_3/1

== system case4/AC_1/d_id_line_1_4_block ==
  note: d_id_line_1_4 in case4
      | $376.991118430775\,\mathrm{iq}_{\mathrm{line},1,4}+6254.53843232971\,\mathrm{vd}_{\mathrm{bus},1}-6254.53843232971\,\mathrm{vd}_{\mathrm{bus},4}$
      | Automatically generated on 2025-10-31 19:07:42 .
  State_iq_line_1_4_0e235 : Inport
  State_vd_bus_1_91d32 : Inport  Port=2
  State_vd_bus_4_3ed23 : Inport  Port=3
  Add_a2548 : Sum
  Constant_376.991118430775_dafdf : Constant  Value=376.991118430775
  Constant_6254.53843232971_2a165 : Constant  Value=6254.53843232971
  Constant_6254.53843232971_579f3 : Constant  Value=6254.53843232971
  Product_8d0d7 : Product
  Product_def34 : Product
  Product_f861d : Product
  Subtract_c9a46 : Sum  Inputs=+-
  Blockout_d_id_line_1_4_c12b1 : Outport
  wires:
  Constant_376.991118430775_dafdf/1 -> Product_8d0d7/1
  Product_f861d/1 -> Add_a2548/2
  State_iq_line_1_4_0e235/1 -> Product_8d0d7/2
  Subtract_c9a46/1 -> Blockout_d_id_line_1_4_c12b1/1
  Constant_6254.53843232971_579f3/1 -> Product_f861d/1
  Product_8d0d7/1 -> Add_a2548/1
  State_vd_bus_1_91d32/1 -> Product_f861d/2
  Constant_6254.53843232971_2a165/1 -> Product_def34/1
  State_vd_bus_4_3ed23/1 -> Product_def34/2
  Add_a2548/1 -> Subtract_c9a46/1
  Product_def34/1 -> Subtract_c9a46/2

== system case4/AC_1/d_id_line_3_6_block ==
  note: d_id_line_3_6 in case4
      | $376.991118430775\,\mathrm{iq}_{\mathrm{line},3,6}+6147.80569457664\,\mathrm{vd}_{\mathrm{bus},3}-6147.80569457664\,\mathrm{vd}_{\mathrm{bus},6}$
      | Automatically generated on 2025-10-31 19:07:49 .
  State_iq_line_3_6_4e988 : Inport
  State_vd_bus_3_a6578 : Inport  Port=2
  State_vd_bus_6_66fef : Inport  Port=3
  Add_9fd59 : Sum
  Constant_376.991118430775_fe2e5 : Constant  Value=376.991118430775
  Constant_6147.80569457664_2f0f3 : Constant  Value=6147.80569457664
  Constant_6147.80569457664_4e39c : Constant  Value=6147.80569457664
  Product_24828 : Product
  Product_5f014 : Product
  Product_a4a99 : Product
  Subtract_e7672 : Sum  Inputs=+-
  Blockout_d_id_line_3_6_d53d7 : Outport
  wires:
  State_vd_bus_3_a6578/1 -> Product_a4a99/2
  Constant_376.991118430775_fe2e5/1 -> Product_24828/1
  Product_a4a99/1 -> Add_9fd59/2
  State_iq_line_3_6_4e988/1 -> Product_24828/2
  Constant_6147.80569457664_4e39c/1 -> Product_a4a99/1
  Product_24828/1 -> Add_9fd59/1
  Constant_6147.80569457664_2f0f3/1 -> Product_5f014/1
  State_vd_bus_6_66fef/1 -> Product_5f014/2
  Add_9fd59/1 -> Subtract_e7672/1
  Product_5f014/1 -> Subtract_e7672/2
  Subtract_e7672/1 -> Blockout_d_id_line_3_6_d53d7/1

== system case4/AC_1/d_id_line_4_5_block ==
  note: d_id_line_4_5 in case4
      | $376.991118430775\,\mathrm{iq}_{\mathrm{line},4,5}-66.2754255159152\,\mathrm{id}_{\mathrm{line},4,5}+3915.88493154556\,\mathrm{vd}_{\mathrm{bus},4}-3915.88493154556\,\mathrm{vd}_{\mathrm{bus},5}$
      | Automatically generated on 2025-10-31 19:07:44 .
  State_id_line_4_5_be8c5 : Inport
  State_iq_line_4_5_1edad : Inport  Port=2
  State_vd_bus_4_de2fb : Inport  Port=3
  State_vd_bus_5_f7ecc : Inport  Port=4
  Add_58046 : Sum
  Add_cedee : Sum
  Constant_-66.2754255159152_35887 : Constant  Value=-66.2754255159152
  Constant_376.991118430775_d86cb : Constant  Value=376.991118430775
  Constant_3915.88493154556_12e34 : Constant  Value=3915.88493154556
  Constant_3915.88493154556_d2060 : Constant  Value=3915.88493154556
  Product_30432 : Product
  Product_a9ff9 : Product
  Product_c8893 : Product
  Product_faa85 : Product
  Subtract_33dcc : Sum  Inputs=+-
  Blockout_d_id_line_4_5_92e48 : Outport
  wires:
  Constant_-66.2754255159152_35887/1 -> Product_faa85/1
  Product_30432/1 -> Add_cedee/2
  State_id_line_4_5_be8c5/1 -> Product_faa85/2
  Constant_376.991118430775_d86cb/1 -> Product_30432/1
  State_iq_line_4_5_1edad/1 -> Product_30432/2
  Product_faa85/1 -> Add_cedee/1
  Constant_3915.88493154556_12e34/1 -> Product_a9ff9/1
  State_vd_bus_4_de2fb/1 -> Product_a9ff9/2
  Add_cedee/1 -> Add_58046/1
  Product_a9ff9/1 -> Add_58046/2
  Constant_3915.88493154556_d2060/1 -> Product_c8893/1
  State_vd_bus_5_f7ecc/1 -> Product_c8893/2
  Add_58046/1 -> Subtract_33dcc/1
  Product_c8893/1 -> Subtract_33dcc/2
  Subtract_33dcc/1 -> Blockout_d_id_line_4_5_92e48/1

== system case4/AC_1/d_id_line_5_6_block ==
  note: d_id_line_5_6 in case4
      | $376.991118430775\,\mathrm{iq}_{\mathrm{line},5,6}-82.282431401766\,\mathrm{id}_{\mathrm{line},5,6}+2119.18478648348\,\mathrm{vd}_{\mathrm{bus},5}-2119.18478648348\,\mathrm{vd}_{\mathrm{bus},6}$
      | Automatically generated on 2025-10-31 19:07:47 .
  State_id_line_5_6_669ed : Inport
  State_iq_line_5_6_e77ce : Inport  Port=2
  State_vd_bus_5_0e564 : Inport  Port=3
  State_vd_bus_6_757cb : Inport  Port=4
  Add_5d23d : Sum
  Add_bebbb : Sum
  Constant_-82.282431401766_4b192 : Constant  Value=-82.282431401766
  Constant_2119.18478648348_6bafe : Constant  Value=2119.18478648348
  Constant_2119.18478648348_b58db : Constant  Value=2119.18478648348
  Constant_376.991118430775_c682e : Constant  Value=376.991118430775
  Product_41a5a : Product
  Product_62401 : Product
  Product_83e06 : Product
  Product_934ab : Product
  Subtract_39d52 : Sum  Inputs=+-
  Blockout_d_id_line_5_6_b7e3f : Outport
  wires:
  Constant_-82.282431401766_4b192/1 -> Product_83e06/1
  Product_41a5a/1 -> Add_5d23d/2
  State_id_line_5_6_669ed/1 -> Product_83e06/2
  Constant_376.991118430775_c682e/1 -> Product_41a5a/1
  Product_83e06/1 -> Add_5d23d/1
  State_iq_line_5_6_e77ce/1 -> Product_41a5a/2
  Constant_2119.18478648348_b58db/1 -> Product_934ab/1
  Product_62401/1 -> Subtract_39d52/2
  State_vd_bus_5_0e564/1 -> Product_934ab/2
  Add_5d23d/1 -> Add_bebbb/1
  Product_934ab/1 -> Add_bebbb/2
  Constant_2119.18478648348_6bafe/1 -> Product_62401/1
  State_vd_bus_6_757cb/1 -> Product_62401/2
  Add_bebbb/1 -> Subtract_39d52/1
  Subtract_39d52/1 -> Blockout_d_id_line_5_6_b7e3f/1

== system case4/AC_1/d_id_line_6_7_block ==
  note: d_id_line_6_7 in case4
      | $376.991118430775\,\mathrm{iq}_{\mathrm{line},6,7}-42.3426329685014\,\mathrm{id}_{\mathrm{line},6,7}+3574.02196133126\,\mathrm{vd}_{\mathrm{bus},6}-3574.02196133126\,\mathrm{vd}_{\mathrm{bus},7}$
      | Automatically generated on 2025-10-31 19:07:52 .
  State_id_line_6_7_205ed : Inport
  State_iq_line_6_7_7334d : Inport  Port=2
  State_vd_bus_6_54d39 : Inport  Port=3
  State_vd_bus_7_0da25 : Inport  Port=4
  Add_3fc1f : Sum
  Add_59719 : Sum
  Constant_-42.3426329685014_cb5d4 : Constant  Value=-42.3426329685014
  Constant_3574.02196133126_01022 : Constant  Value=3574.02196133126
  Constant_3574.02196133126_e9647 : Constant  Value=3574.02196133126
  Constant_376.991118430775_3f74d : Constant  Value=376.991118430775
  Product_2b39d : Product
  Product_45d08 : Product
  Product_686c8 : Product
  Product_74d33 : Product
  Subtract_ea645 : Sum  Inputs=+-
  Blockout_d_id_line_6_7_bd2cf : Outport
  wires:
  Constant_-42.3426329685014_cb5d4/1 -> Product_74d33/1
  Product_686c8/1 -> Add_59719/2
  State_id_line_6_7_205ed/1 -> Product_74d33/2
  Constant_376.991118430775_3f74d/1 -> Product_686c8/1
  State_iq_line_6_7_7334d/1 -> Product_686c8/2
  Product_74d33/1 -> Add_59719/1
  Constant_3574.02196133126_01022/1 -> Product_45d08/1
  State_vd_bus_6_54d39/1 -> Product_45d08/2
  Add_59719/1 -> Add_3fc1f/1
  Product_45d08/1 -> Add_3fc1f/2
  Constant_3574.02196133126_e9647/1 -> Product_2b39d/1
  State_vd_bus_7_0da25/1 -> Product_2b39d/2
  Add_3fc1f/1 -> Subtract_ea645/1
  Product_2b39d/1 -> Subtract_ea645/2
  Subtract_ea645/1 -> Blockout_d_id_line_6_7_bd2cf/1

== system case4/AC_1/d_id_line_7_8_block ==
  note: d_id_line_7_8 in case4
      | $376.991118430775\,\mathrm{iq}_{\mathrm{line},7,8}-42.3426329685014\,\mathrm{id}_{\mathrm{line},7,8}+5003.63074586377\,\mathrm{vd}_{\mathrm{bus},7}-5003.63074586377\,\mathrm{vd}_{\mathrm{bus},8}$
      | Automatically generated on 2025-10-31 19:07:54 .
  State_id_line_7_8_95bec : Inport
  State_iq_line_7_8_b5b80 : Inport  Port=2
  State_vd_bus_7_dfa37 : Inport  Port=3
  State_vd_bus_8_a71c0 : Inport  Port=4
  Add_7973c : Sum
  Add_bb054 : Sum
  Constant_-42.3426329685014_30eb1 : Constant  Value=-42.3426329685014
  Constant_376.991118430775_8ed03 : Constant  Value=376.991118430775
  Constant_5003.63074586377_92db0 : Constant  Value=5003.63074586377
  Constant_5003.63074586377_cbedd : Constant  Value=5003.63074586377
  Product_1feee : Product
  Product_50ad5 : Product
  Product_964cc : Product
  Product_a4905 : Product
  Subtract_098d0 : Sum  Inputs=+-
  Blockout_d_id_line_7_8_fa870 : Outport
  wires:
  Constant_-42.3426329685014_30eb1/1 -> Product_964cc/1
  Product_50ad5/1 -> Add_bb054/2
  State_id_line_7_8_95bec/1 -> Product_964cc/2
  Constant_376.991118430775_8ed03/1 -> Product_50ad5/1
  Product_964cc/1 -> Add_bb054/1
  State_iq_line_7_8_b5b80/1 -> Product_50ad5/2
  Constant_5003.63074586377_cbedd/1 -> Product_1feee/1
  State_vd_bus_7_dfa37/1 -> Product_1feee/2
  Add_bb054/1 -> Add_7973c/1
  Product_1feee/1 -> Add_7973c/2
  Constant_5003.63074586377_92db0/1 -> Product_a4905/1
  State_vd_bus_8_a71c0/1 -> Product_a4905/2
  Add_7973c/1 -> Subtract_098d0/1
  Product_a4905/1 -> Subtract_098d0/2
  Subtract_098d0/1 -> Blockout_d_id_line_7_8_fa870/1

== system case4/AC_1/d_id_line_8_2_block ==
  note: d_id_line_8_2 in case4
      | $376.991118430775\,\mathrm{iq}_{\mathrm{line},8,2}-5764.18261923506\,\mathrm{vd}_{\mathrm{bus},2}+5764.18261923506\,\mathrm{vd}_{\mathrm{bus},8}$
      | Automatically generated on 2025-10-31 19:07:56 .
  State_iq_line_8_2_fc8b9 : Inport
  State_vd_bus_2_f74f3 : Inport  Port=2
  State_vd_bus_8_bcd3f : Inport  Port=3
  Add_14330 : Sum
  Constant_376.991118430775_edb39 : Constant  Value=376.991118430775
  Constant_5764.18261923506_5839c : Constant  Value=5764.18261923506
  Constant_5764.18261923506_ef04b : Constant  Value=5764.18261923506
  Product_24f28 : Product
  Product_2d929 : Product
  Product_5bc6c : Product
  Subtract_a0b37 : Sum  Inputs=+-
  Blockout_d_id_line_8_2_d5ea8 : Outport
  wires:
  State_vd_bus_2_f74f3/1 -> Product_2d929/2
  Constant_376.991118430775_edb39/1 -> Product_5bc6c/1
  Product_2d929/1 -> Subtract_a0b37/2
  State_iq_line_8_2_fc8b9/1 -> Product_5bc6c/2
  Constant_5764.18261923506_5839c/1 -> Product_2d929/1
  Product_5bc6c/1 -> Subtract_a0b37/1
  Constant_5764.18261923506_ef04b/1 -> Product_24f28/1
  State_vd_bus_8_bcd3f/1 -> Product_24f28/2
  Subtract_a0b37/1 -> Add_14330/1
  Product_24f28/1 -> Add_14330/2
  Add_14330/1 -> Blockout_d_id_line_8_2_d5ea8/1

== system case4/AC_1/d_id_line_8_9_block ==
  note: d_id_line_8_9 in case4
      | $376.991118430775\,\mathrm{iq}_{\mathrm{line},8,9}-71.2878526557744\,\mathrm{id}_{\mathrm{line},8,9}+2237.64853231175\,\mathrm{vd}_{\mathrm{bus},8}-2237.64853231175\,\mathrm{vd}_{\mathrm{bus},9}$
      | Automatically generated on 2025-10-31 19:07:59 .
  State_id_line_8_9_d1adb : Inport
  State_iq_line_8_9_5adad : Inport  Port=2
  State_vd_bus_8_62172 : Inport  Port=3
  State_vd_bus_9_f74b0 : Inport  Port=4
  Add_366fc : Sum
  Add_c4554 : Sum
  Constant_-71.2878526557744_85d18 : Constant  Value=-71.2878526557744
  Constant_2237.64853231175_65e52 : Constant  Value=2237.64853231175
  Constant_2237.64853231175_a5b29 : Constant  Value=2237.64853231175
  Constant_376.991118430775_4fe42 : Constant  Value=376.991118430775
  Product_42a1f : Product
  Product_843db : Product
  Product_9821e : Product
  Product_c874a : Product
  Subtract_eec8f : Sum  Inputs=+-
  Blockout_d_id_line_8_9_12877 : Outport
  wires:
  Constant_-71.2878526557744_85d18/1 -> Product_9821e/1
  Product_843db/1 -> Add_366fc/2
  State_id_line_8_9_d1adb/1 -> Product_9821e/2
  Constant_376.991118430775_4fe42/1 -> Product_843db/1
  State_iq_line_8_9_5adad/1 -> Product_843db/2
  Product_9821e/1 -> Add_366fc/1
  Constant_2237.64853231175_a5b29/1 -> Product_42a1f/1
  State_vd_bus_8_62172/1 -> Product_42a1f/2
  Add_366fc/1 -> Add_c4554/1
  Product_42a1f/1 -> Add_c4554/2
  Constant_2237.64853231175_65e52/1 -> Product_c874a/1
  State_vd_bus_9_f74b0/1 -> Product_c874a/2
  Add_c4554/1 -> Subtract_eec8f/1
  Product_c874a/1 -> Subtract_eec8f/2
  Subtract_eec8f/1 -> Blockout_d_id_line_8_9_12877/1

== system case4/AC_1/d_id_line_9_4_block ==
  note: d_id_line_9_4 in case4
      | $376.991118430775\,\mathrm{iq}_{\mathrm{line},9,4}-42.1961186675723\,\mathrm{id}_{\mathrm{line},9,4}-4238.36957296695\,\mathrm{vd}_{\mathrm{bus},4}+4238.36957296695\,\mathrm{vd}_{\mathrm{bus},9}$
      | Automatically generated on 2025-10-31 19:08:01 .
  State_id_line_9_4_a375b : Inport
  State_iq_line_9_4_d03ba : Inport  Port=2
  State_vd_bus_4_18861 : Inport  Port=3
  State_vd_bus_9_95759 : Inport  Port=4
  Add_91de8 : Sum
  Add_9630b : Sum
  Constant_-42.1961186675723_ca432 : Constant  Value=-42.1961186675723
  Constant_376.991118430775_3cfcf : Constant  Value=376.991118430775
  Constant_4238.36957296695_842f3 : Constant  Value=4238.36957296695
  Constant_4238.36957296695_b732b : Constant  Value=4238.36957296695
  Product_27acb : Product
  Product_b2c9e : Product
  Product_b572c : Product
  Product_d11ca : Product
  Subtract_3c20b : Sum  Inputs=+-
  Blockout_d_id_line_9_4_11d37 : Outport
  wires:
  Constant_-42.1961186675723_ca432/1 -> Product_b572c/1
  Product_b2c9e/1 -> Add_9630b/2
  State_id_line_9_4_a375b/1 -> Product_b572c/2
  Constant_376.991118430775_3cfcf/1 -> Product_b2c9e/1
  Product_b572c/1 -> Add_9630b/1
  State_iq_line_9_4_d03ba/1 -> Product_b2c9e/2
  Constant_4238.36957296695_b732b/1 -> Product_27acb/1
  State_vd_bus_4_18861/1 -> Product_27acb/2
  Add_9630b/1 -> Subtract_3c20b/1
  Product_27acb/1 -> Subtract_3c20b/2
  Constant_4238.36957296695_842f3/1 -> Product_d11ca/1
  Subtract_3c20b/1 -> Add_91de8/1
  State_vd_bus_9_95759/1 -> Product_d11ca/2
  Product_d11ca/1 -> Add_91de8/2
  Add_91de8/1 -> Blockout_d_id_line_9_4_11d37/1

== system case4/AC_1/d_id_load_5_block ==
  note: d_id_load_5 in case4
      | $376.991118430775\,\mathrm{iq}_{\mathrm{load},5}-1079.91892759499\,\mathrm{id}_{\mathrm{load},5}+1157.47551177004\,\mathrm{vd}_{\mathrm{bus},5}$
      | Automatically generated on 2025-10-31 19:07:36 .
  State_id_load_5_45f50 : Inport
  State_iq_load_5_dfbd7 : Inport  Port=2
  State_vd_bus_5_078f0 : Inport  Port=3
  Add_f49dd : Sum
  Add_f83dd : Sum
  Constant_-1079.91892759499_87f19 : Constant  Value=-1079.91892759499
  Constant_1157.47551177004_60e16 : Constant  Value=1157.47551177004
  Constant_376.991118430775_5f2d7 : Constant  Value=376.991118430775
  Product_1a414 : Product
  Product_36533 : Product
  Product_b3590 : Product
  Blockout_d_id_load_5_3ae5a : Outport
  wires:
  Constant_-1079.91892759499_87f19/1 -> Product_1a414/1
  Product_36533/1 -> Add_f49dd/2
  State_id_load_5_45f50/1 -> Product_1a414/2
  Constant_376.991118430775_5f2d7/1 -> Product_36533/1
  Product_b3590/1 -> Add_f83dd/2
  State_iq_load_5_dfbd7/1 -> Product_36533/2
  Product_1a414/1 -> Add_f49dd/1
  Constant_1157.47551177004_60e16/1 -> Product_b3590/1
  State_vd_bus_5_078f0/1 -> Product_b3590/2
  Add_f49dd/1 -> Add_f83dd/1
  Add_f83dd/1 -> Blockout_d_id_load_5_3ae5a/1
